simulink model "leadCompensatorSimulation_v2"  (R2023b)
settings: Solver=VariableStepAuto  StartTime=0  StopTime=1.712  RelTol=1e-3
values from neighbouring files (symbols this model uses):
  ad = exp(-T_sample*pd_param.a)    [measureFrequencyResponse.m]    (also in measureFrequencyResponse_pd.m = exp(-Ts*pd_param.a))
  b = 0.010585    [init.m]    (also in system_parameters.mat = 0.0078)
  dc_minus = -0.3201    [init.m]    (also in system_parameters.mat = -0.5)
  dc_plus = 0.34    [init.m]    (also in system_parameters.mat = 0.5)
  delta_x = 4.63e-04    (= 0.000463)    [init.m]    (also in system_parameters.mat = 0.02)
  enableSimModelFriction = true    [measureFrequencyResponse.m]    (also in measureFrequencyResponse_pd.m)
  Kd = Kp*(Td-Ta)    [designPD_lead_compensator.m]    (also in designPID_lead_compensator.m = K*(Ti-Ta)*(Td-Ta); measureFrequencyResponse.m = pd_param.Kd; measureFrequencyResponse_pd.m = pd_param.Kd)
  Ki = K    [designPID_lead_compensator.m]    (also in measureFrequencyResponse.m = pd_param.Ki; measureFrequencyResponse_pd.m = pd_param.Ki)
  Kp = abs(j*w_c*Ta + 1)/( abs(j*w_c*Td + 1) * mag_G_jwc)    [designLeadCompensator.m]    (also in designPD_lead_compensator.m = lc_param.Kp; designPID_lead_compensator.m = K*(Ti+Td-Ta); measureFrequencyResponse.m = pd_param.Kp; measureFrequencyResponse_pd.m = pd_param.Kp)
  m = 6.8930e-04    (= 0.0006893)    [init.m]    (also in system_parameters.mat)
  Ts = 0.001    [init.m]    (also in measureFrequencyResponse.m; measureFrequencyResponse_pd.m; system_parameters.mat)
undefined symbols (not defined in the file or in its folder): DiscIntNeverNeededParam
libraries: simulink x1
settings Model: Creator=sanjeevsapkota271828
settings SolverCC: ZeroCrossAlgorithm=Adaptive
settings DebuggingCC: IgnoredZcDiagnostic=none  UnconnectedInputMsg=warning  UnconnectedOutputMsg=warning  UnconnectedLineMsg=warning
settings ModelReferenceCC: EnableRefExpFcnMdlSchedulingChecks=on
settings RTWCC: DLArmComputeVersion=19.05

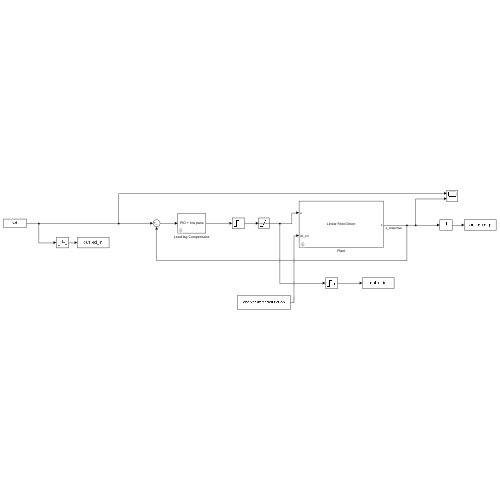
[thumbnail: Simulink's stored preview of the top-level diagram]
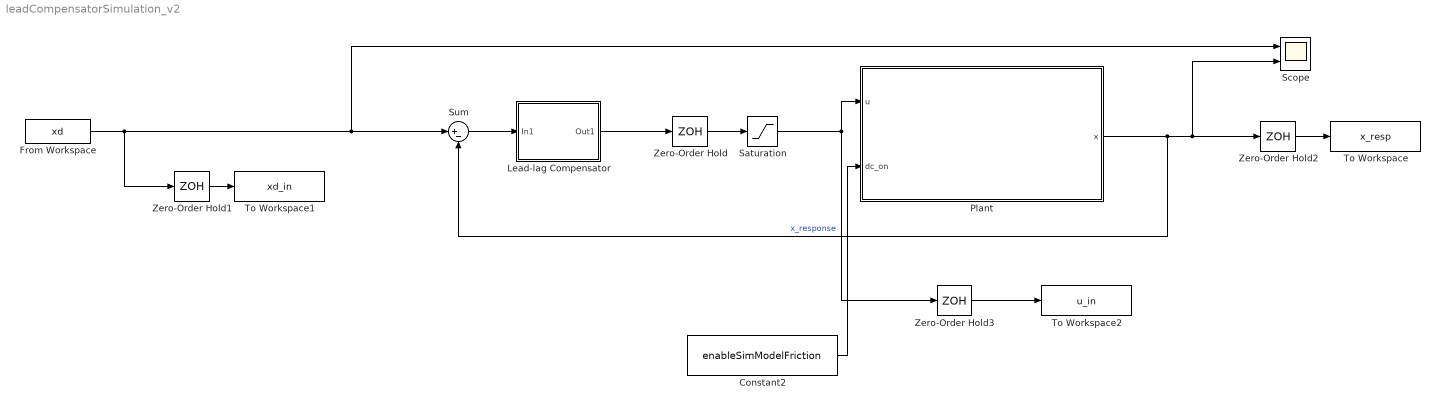
== system leadCompensatorSimulation_v2 ==
  Constant2 : Constant  Value=enableSimModelFriction
  From Workspace : FromWorkspace  VariableName=xd
  Lead-lag Compensator : Subsystem  mask{kp=Kp, ki=Ki, kd=Kd, ad=ad}
      mask Display: disp("PID + low pass")
  Plant : Subsystem  mask{m=m, b=b, dc_p=dc_plus, dc_m=dc_minus, delta_x=delta_x}
      mask prompts: m "mass"; b "damping"; dc_p "coloumb friction [forward]"; dc_m "coloumb friction [backward]"
      mask DialogControl DescGroupVar Prompt: Rack and pinion feed drive
      mask DialogControl DescTextVar Prompt: Computes dynamics and returns quantized data as input
      mask Display: disp("Linear Feed Drive:")
  Saturation : Saturate  UpperLimit=3.5  LowerLimit=-3.5
  Scope : Scope  NumInputPorts=2
  Sum : Sum  Inputs=|+-
  To Workspace : ToWorkspace  VariableName=x_resp  SaveFormat=Structure With Time  SampleTime=-1
  To Workspace1 : ToWorkspace  VariableName=xd_in  SaveFormat=Structure With Time  SampleTime=-1
  To Workspace2 : ToWorkspace  VariableName=u_in  SaveFormat=Structure With Time  SampleTime=-1
  Zero-Order Hold{,1..3} (4 alike) : ZeroOrderHold  SampleTime=Ts
  wires:
  Saturation/1 -> Zero-Order Hold3/1, Plant/1(u)
  Sum/1 -> Lead-lag Compensator/1(In1)
  Constant2/1 -> Plant/2(dc_on)
  Lead-lag Compensator/1(Out1) -> Zero-Order Hold/1
  Zero-Order Hold/1 -> Saturation/1
  Plant/1(x) -> Sum/2, Scope/2, Zero-Order Hold2/1  "x_response"
  From Workspace/1 -> Zero-Order Hold1/1, Scope/1, Sum/1
  Zero-Order Hold1/1 -> To Workspace1/1
  Zero-Order Hold2/1 -> To Workspace/1
  Zero-Order Hold3/1 -> To Workspace2/1

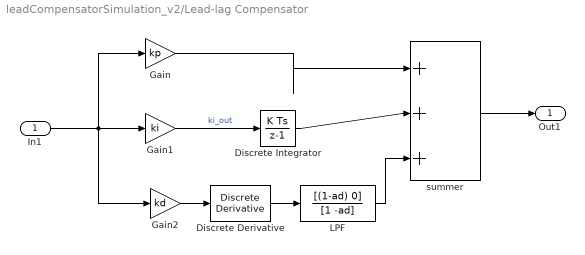
== system leadCompensatorSimulation_v2/Lead-lag Compensator ==
  In1 : Inport
  Discrete Derivative : simulink/Discrete/Discrete Derivative  gainval=1.0  ICPrevScaledInput=0.0  OutMin=[]  OutMax=[]  OutDataType=fixdt(1, 16)  OutScaling=2^-10  DoSatur=off
  Discrete Integrator : DiscreteIntegrator  SampleTime=Ts  ICPrevOutput=DiscIntNeverNeededParam  ICPrevScaledInput=DiscIntNeverNeededParam
  Gain : Gain  Gain=kp
  Gain1 : Gain  Gain=ki
  Gain2 : Gain  Gain=kd
  LPF : DiscreteTransferFcn  Numerator=[(1-ad) 0]  Denominator=[1 -ad]
  summer : Sum  Inputs=|+++
  Out1 : Outport
  wires:
  In1/1 -> Gain2/1, Gain1/1, Gain/1
  summer/1 -> Out1/1
  Gain/1 -> summer/1
  Gain1/1 -> Discrete Integrator/1  "ki_out"
  Discrete Integrator/1 -> summer/2
  Gain2/1 -> Discrete Derivative/1
  Discrete Derivative/1 -> LPF/1
  LPF/1 -> summer/3

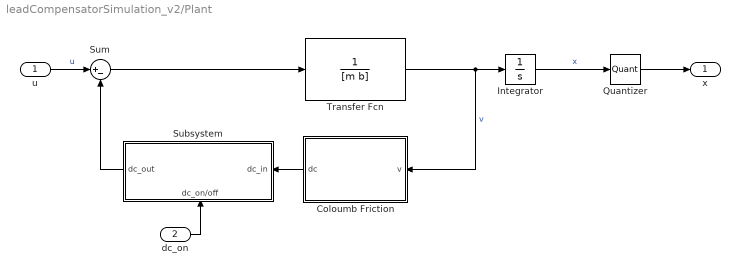
== system leadCompensatorSimulation_v2/Plant ==
  u : Inport
  dc_on : Inport  Port=2
  Coloumb Friction : Subsystem  mask{dc_p=dc_p, dc_m=dc_m}
      mask prompts: dc_p "forward friction"; dc_m "backward friction"
      settings: PortSchema="{\"entries\":[{\"content\":{\"sides\":[{\"content\":{\"connectorIds\":[\"Out1\"]},\"type\":\"ConnectorPlacement.EquallySpacedRectSide\",\"uuid\":\"ff12b2c0-96a7-455e-a8b4-07c6e260c366\"},{\"content\":{\"connectorIds\":[\"In1\"],\"side\":\"RIGHT\"},\"type\":\"ConnectorPlacement.EquallySpacedRectSide\",\"uuid\":\"07b26d63-6ebc-42e8-853f-da6a99fdc545\"},{\"content\":{\"connectorIds\":[],\"side\":\"TOP\"},\"type\":\"ConnectorPlacement.EquallySpacedRectSide\",\"uuid\":\"d2c0cb8d-d4ca-4771-a065-4043ea3005cf\"},{\"content\":{\"connectorIds\":[],\"side\":\"BOTTOM\"},\"type\":\"ConnectorPlacement.EquallySpacedRectSide\",\"uuid\":\"2ea35cc4-4f9d-416c-aca4-3e26f4283c75\"}]},\"type\":\"ConnectorPlacement.EquallySpacedConnector\",\"uuid\":\"16e67640-52fd-406f-b94d-ae51e9d687b6\"}],\"packageUris\":[\"http://schema.mathworks.com/mf0/Connector/R2020b\"],\"version\":\"1.0\"}"
      mask DialogControl DescGroupVar Prompt: Coloumb Friction
      mask Display:
      | % f(u)
      | disp("Coloumb Friction")
  Integrator : Integrator
  Quantizer : Quantizer  QuantizationInterval=delta_x
  Subsystem : Subsystem
      settings: PortSchema="{\"entries\":[{\"content\":{\"sides\":[{\"content\":{\"connectorIds\":[\"Out1\"]},\"type\":\"ConnectorPlacement.EquallySpacedRectSide\",\"uuid\":\"ff12b2c0-96a7-455e-a8b4-07c6e260c366\"},{\"content\":{\"connectorIds\":[\"In2\"],\"side\":\"RIGHT\"},\"type\":\"ConnectorPlacement.EquallySpacedRectSide\",\"uuid\":\"07b26d63-6ebc-42e8-853f-da6a99fdc545\"},{\"content\":{\"connectorIds\":[],\"side\":\"TOP\"},\"type\":\"ConnectorPlacement.EquallySpacedRectSide\",\"uuid\":\"d2c0cb8d-d4ca-4771-a065-4043ea3005cf\"},{\"content\":{\"connectorIds\":[\"In1\"],\"side\":\"BOTTOM\"},\"type\":\"ConnectorPlacement.EquallySpacedRectSide\",\"uuid\":\"15ad21a6-a752-41a3-ac9c-d8a20b0e6199\"}]},\"type\":\"ConnectorPlacement.EquallySpacedConnector\",\"uuid\":\"16e67640-52fd-406f-b94d-ae51e9d687b6\"}],\"packageUris\":[\"http://schema.mathworks.com/mf0/Connector/R2020b\"],\"version\":\"1.0\"}"
  Sum : Sum  Inputs=|+-
  Transfer Fcn : TransferFcn  Denominator=[m b]
  x : Outport
  wires:
  Transfer Fcn/1 -> Coloumb Friction/1(v), Integrator/1  "v"
  u/1 -> Sum/1  "u"
  Sum/1 -> Transfer Fcn/1
  Integrator/1 -> Quantizer/1  "x"
  Quantizer/1 -> x/1
  Coloumb Friction/1(dc) -> Subsystem/2(dc_in)
  Subsystem/1(dc_out) -> Sum/2
  dc_on/1 -> Subsystem/1(dc_on/off)

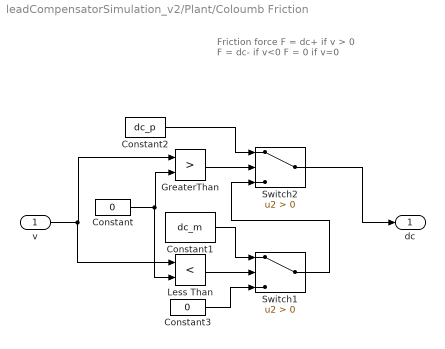
== system leadCompensatorSimulation_v2/Plant/Coloumb Friction ==
  note: Friction force
      | F = dc+ if v > 0
      | F = dc- if v<0
      | F = 0 if v=0
  v : Inport
  Constant : Constant  Value=0
  Constant1 : Constant  Value=dc_m
  Constant2 : Constant  Value=dc_p
  Constant3 : Constant  Value=0
  GreaterThan : RelationalOperator  Operator=>  OutDataTypeStr=boolean  RndMeth=Simplest  InputSameDT=off
  Less Than : RelationalOperator  Operator=<  OutDataTypeStr=boolean  RndMeth=Simplest  InputSameDT=off
  Switch1 : Switch  Criteria=u2 > Threshold  SaturateOnIntegerOverflow=off  InputSameDT=off
  Switch2 : Switch  Criteria=u2 > Threshold  SaturateOnIntegerOverflow=off  InputSameDT=off
  dc : Outport
  wires:
  GreaterThan/1 -> Switch2/2
  Constant/1 -> Less Than/2, GreaterThan/2
  Less Than/1 -> Switch1/2
  v/1 -> Less Than/1, GreaterThan/1
  Switch1/1 -> Switch2/3
  Constant1/1 -> Switch1/1
  Constant2/1 -> Switch2/1
  Switch2/1 -> dc/1
  Constant3/1 -> Switch1/3

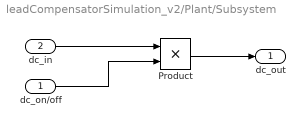
== system leadCompensatorSimulation_v2/Plant/Subsystem ==
  dc_on/off : Inport
  dc_in : Inport  Port=2
  Product : Product
  dc_out : Outport
  wires:
  dc_in/1 -> Product/1
  dc_on/off/1 -> Product/2
  Product/1 -> dc_out/1
